simulink model "HMC"  (R2026a)
settings: Solver=ode1  StopTime=inf  FixedStep=0.0001
PreLoadFcn:
  | %load('C:\Users\bme_master\Desktop\mot\mot_6_deneme.mat')
  | 
  | 
  | %load('C:\Users\bme_master\Desktop\mot\PRE_G''s.mat')
PostLoadFcn:
  | , if any(exist('dsrtsu_mdlpostloadfcn', 'file') ~= 0), dsrtsu_mdlpostloadfcn('Execute', bdroot); end,
InitFcn:
  | %motor_control_init_m
  | %clear all
  | %close all
  | %clc
  | b=1e-8
  | StepSize = 1e-4;
  | N=1e-17;
  | 
  | VLV_0 =0;%120; %120
  | VA_0 = 0;%300; %300
  | VRV_0 = 0;%130;
  | VP_0 = 0;%500;
  | VLA_0 = 0;%20;
  | VV_0=5000;
  | VRA_0=0;
  | 
  | 
  | QLV_0 = 0;
  | QLA_0 = 0;
  | QP_0 = 0;
  | 
  | bh = 0;
  | th =0;
  | 
  | X_0 = [VLV_0 VA_0 VV_0 VP_0  VLA_0  VRA_0 VRV_0];
  | 
  | 
  | V0 = 10;
  | 
  | K1=.0004;%0.0001
  | K2=0.0009;%0.0009
  | KA=1;%1
  | C1=0.000000003;%0.0000003
  | lambda=6000;%3000
  | X_00 = [VLV_0 VA_0 VV_0 VRV_0];
  | 
  | r2 = 0.05/2;
  | A2 = pi*r2^2;
  | h2 = 0.63;
  | V2 = A2*h2;
  | 
  | 
  | r3 = 0.05/2;
  | A3 = pi*r3^2;
  | h3 = 0.63;
  | V3 = A3*h3;
  | 
  | 
  | rho = 997;
  | gg = 9.81;
  | %
  | init_min=0;
  | init_max=0;
  | %
  | PWM_Period =  StepSize;
  | PWM_Period_g1 = PWM_Period;
  | PWM_Period_g2 =PWM_Period;
  | PWM_Period_g3 = PWM_Period;
  | PWM_Period_g4 = PWM_Period;
  | PWM_Period_g5 = PWM_Period;
  | ... (+158 lines)
undefined symbols (not defined in the file or in its folder): Continuous, DiscIntNeverNeededParam, Time
libraries: powerlib_meascontrol x19, simulink x15, rti1202lib_adc_class1 x11, cstblocks x10, rti1202lib_dio_class1 x8, dspstat3 x3, rti1202lib_dac_class1 x1, dspswit3 x1, ctrlSharedLib x1, slpidlib x1, dsparch4 x1
(part 2 of 5)

== system HMC/DP_calc ==
  Subtract : Sum  Inputs=+-
  Out1 : Outport  VectorParamsAs1DForOutWhenUnconnected=off
  wires:
  [P2_mmHg] -> Subtract/1
  [P3_mmHg] -> Subtract/2
  Subtract/1 -> Out1/1

== system HMC/DV_calc ==
  DV : Scope
      settings: DataLoggingVariableName=ScopeData7
  MATLAB Function3 : MATLAB Function  TreatAsAtomicUnit=on
  Transfer Fcn1 : TransferFcn  Numerator=[100^2]  Denominator=[1 2*5*100 100^2]
  V2 : Scope
      settings: DataLoggingVariableName=ScopeData5
  V3 : Scope
      settings: DataLoggingVariableName=ScopeData6
  Out1 : Outport  VectorParamsAs1DForOutWhenUnconnected=off
  wires:
  [P2_Pa] -> MATLAB Function3/1(P2)
  MATLAB Function3/1(V2) -> V2/1
  [P3_Pa] -> MATLAB Function3/3(P3)
  [P2p_Pa] -> MATLAB Function3/2(Pp2)
  MATLAB Function3/2(V3) -> V3/1
  [P3p_Pa] -> MATLAB Function3/4(Pp3)
  MATLAB Function3/3(DV) -> Transfer Fcn1/1
  Transfer Fcn1/1 -> DV/1, Out1/1

== system HMC/IBS_LVAD ==
  Subsystem1 : Subsystem
  Unit Delay : UnitDelay  SampleTime=-1
  W : Outport  VectorParamsAs1DForOutWhenUnconnected=off
  tag scope: VAD_real=global
  wires:
  [x_pre_1] -> Subsystem1/11(VLV)
  [VAD] -> Subsystem1/10(QVAD)
  Unit Delay/1 -> [VAD_real]
  [gLV] -> Subsystem1/18(gLV)
  [PA] -> Subsystem1/20(PA1)
  Subsystem1/1(VAD) -> Unit Delay/1
  [eLV] -> Subsystem1/15(eLV)
  [eRA] -> Subsystem1/12(eRA)
  [QA] -> Subsystem1/7(QA)
  [PA] -> Subsystem1/2(PA)
  [PLV] -> Subsystem1/19(PLV1)
  [eV] -> Subsystem1/14(eV)
  [PRA] -> Subsystem1/4(PRA)
  [eAO] -> Subsystem1/13(eA)
  [gAO] -> Subsystem1/16(gA)
  [QV] -> Subsystem1/8(QV)
  [gV] -> Subsystem1/17(gV)
  [QLV] -> Subsystem1/6(QLV)
  [PV] -> Subsystem1/3(PV)
  [QLA] -> Subsystem1/5(QLA)
  [PLV] -> Subsystem1/1(PLV)
  [QRA] -> Subsystem1/9(QRA)
  Subsystem1/2(W) -> W/1

== system HMC/KALMAN 3 STATES PLA ==
  Constant7 : Constant  Value=[1 0 0;0 1 0]
  Constant8 : Constant  Value=[0;0]  VectorParams1D=off
  Demux5 : Demux  Outputs=3
  Derivative : Derivative
  Kalman Filter : ctrlSharedLib/Kalman Filter  TimeDomain=Continuous-Time  UseCurrentEstimator=on  ModelSource=Input port  ModelSourceVariable=ss(0.95,1,1,0,1)  A=0.95  B=1  C=1  D=0  NumberOfStates=3  NumberOfInputs=1  NumberOfOutputs=2  InitialEstimateSource=Dialog  X0=[100 0 0]  P0=[1e-2 1e-2 1e-5]  UseK=off  UseGH=off  NumberOfProcessNoiseInputs=1  G=1  TimeInvariantG=on  H=0  TimeInvariantH=on  Q=[100 100 1e-5]  TimeInvariantQ=on  R=[1e-6 1e-5]  TimeInvariantR=on  N=0  TimeInvariantN=on  AddInputPort=on  AddEnablePort=off  OutputEstimatedY=off  OutputP=off  Ts=-1
  MATLAB Function1 : MATLAB Function  TreatAsAtomicUnit=on
  MATLAB Function9 : MATLAB Function  TreatAsAtomicUnit=on
  Mux5 : Mux  Inputs=2
  Mux6 : Mux  Inputs=7
  Scope10 : Scope  NumInputPorts=2
      settings: ActiveDisplayYMinimum=50.21546  ActiveDisplayYMaximum=84.01485
  Scope12 : Scope  NumInputPorts=2
      settings: ActiveDisplayYMinimum=-39.55497  ActiveDisplayYMaximum=141.8795  DataLoggingVariableName=ScopeData2
  Scope13 : Scope  NumInputPorts=2
      settings: ActiveDisplayYMinimum=10.94345  ActiveDisplayYMaximum=14.67296  DataLoggingVariableName=ScopeData3
  Output : Outport  VectorParamsAs1DForOutWhenUnconnected=off
  wires:
  [PA] -> Scope10/2
  Demux5/3 -> Scope13/1, [estPLA], Output/1  "EST PLA"
  Mux5/1 -> Kalman Filter/2
  [PLA] -> Scope13/2
  [eLA] -> Mux6/6
  [PLV] -> Mux5/2
  MATLAB Function9/1(y) -> Kalman Filter/4
  Constant8/1 -> Kalman Filter/6
  [eAO] -> Mux6/4
  [eLV] -> Derivative/1, Mux6/1
  [PA] -> Mux5/1
  Mux6/1 -> MATLAB Function9/1(u), MATLAB Function1/1(u)
  [estPLA] -> MATLAB Function1/3(pla)
  [gLA] -> Mux6/7
  [V0] -> Kalman Filter/1
  Derivative/1 -> Mux6/2
  Demux5/1 -> Scope10/1
  Constant7/1 -> Kalman Filter/5
  Demux5/2 -> Scope12/1
  MATLAB Function1/1(y) -> Kalman Filter/3
  [PLV] -> MATLAB Function1/2(plv)
  [gLV] -> Mux6/3
  Kalman Filter/1 -> Demux5/1
  [PLV] -> Scope12/2
  [gAO] -> Mux6/5

== system HMC/RTI Data ==
  RTI Data Store : Subsystem  Tag=struct('private',struct('version',struct('dsVer',uint32(2)),'access',struct('modified',['21-Nov-2025 12:44:49'],'type','Model','isPerm',1)))  mask(RTI_DATA_STORE){}
      mask help:
      | RTI Data Store Block. This block is used by RTI to store internal model dependent data. Deleting this block will result in data loss.
      |
      | NEVER DELETE, COPY, OR MODIFY THIS BLOCK!
      mask Help:
      | RTI Data Store Block. This block is used by RTI to store internal model dependent data. Deleting this block will result in data loss.
      | 
      | NEVER DELETE, COPY, OR MODIFY THIS BLOCK!
      mask Display: text(0.5, 0.5, ' ', 'HorizontalAlignment', 'center');

== system HMC/Real_IBS ==
  A1 : Constant  Value=0.000234
  A2 : Constant  Value=500
  A3 : Constant  Value=1249
  A4 : Constant  Value=62584000
  Add : Sum
  Add1 : Sum  Inputs=+-
  Constant : Constant  Value=0.3682
  Delta_P1 : Gain
  EQ : Subsystem  Commented=on
  EV_int_scope : Scope
      settings: DataLoggingVariableName=ScopeData4
  EV_scope : Scope
      settings: DataLoggingVariableName=ScopeData5
  Gain : Gain  Gain=1/24
  Gain1 : Gain  Gain=0.0001
  Integrator1 : Integrator  ExternalReset=rising
  J : Constant  Value=1E-05
  K3 : Constant  Value=0.001
  K4 : Constant  Value=0.001
  KV : Constant  Value=20
  MATLAB Function1 : MATLAB Function  TreatAsAtomicUnit=on
  Memory : Memory  InitialCondition=1
  Mux1 : Mux
  Q_vad_dot1 : Subsystem  Commented=on
  Referance_Delta_V_dot : Constant  Value=0
  Subsystem2 : Subsystem
  Subsystem3 : Subsystem  Commented=on
  Subtract : Sum  Inputs=+-
  Transfer Fcn : TransferFcn  Numerator=[100^2]  Denominator=[1 2*5*100 100^2]
  Transfer Fcn1 : TransferFcn  Numerator=[100^2]  Denominator=[1 2*5*100 100^2]
  alpha_P : Constant  Value=2.34E-07
  alpha_Q : Constant  Value=2E-05
  kv : Constant  Value=0.001
  lambda : Constant  Value=0.1
  y_Scope : Scope
      settings: ActiveDisplayYMinimum=-7.21272180033628E+9  ActiveDisplayYMaximum=8.0141354018687E+8  DataLoggingVariableName=ScopeData3
  Out1 : Outport  VectorParamsAs1DForOutWhenUnconnected=off
  wires:
  MATLAB Function1/1(v) -> Gain/1, y_Scope/1
  Gain/1 -> Transfer Fcn/1
  [C_on_off] -> Integrator1/2
  Integrator1/1 -> EV_int_scope/1, MATLAB Function1/10(EV_int)
  Subsystem2/1(Out1) -> Transfer Fcn1/1
  Delta_P1/1 -> MATLAB Function1/7(DP)
  kv/1 -> MATLAB Function1/6(kv)
  KV/1 -> MATLAB Function1/5(KV)
  lambda/1 -> MATLAB Function1/4(lambda)
  J/1 -> MATLAB Function1/3(J)
  alpha_P/1 -> MATLAB Function1/2(alpha_P)
  alpha_Q/1 -> MATLAB Function1/1(alpha_Q)
  [P3_mmHg] -> Subtract/2
  Constant/1 -> Add/2
  Add/1 -> Delta_P1/1
  [P2_mmHg] -> Subtract/1
  Subtract/1 -> Add/1
  Memory/1 -> Add1/2
  [Qvad_kalman] -> Add1/1, Memory/1
  Add1/1 -> Gain1/1
  Gain1/1 -> MATLAB Function1/8(Q_vad_dot)
  K3/1 -> MATLAB Function1/11(K3)
  K4/1 -> MATLAB Function1/12(K4)
  [Qvad_kalman] -> MATLAB Function1/14(Q_vad)
  [Qgp_kalman] -> MATLAB Function1/15(Q_gp)
  Referance_Delta_V_dot/1 -> MATLAB Function1/13(DV_dot_ref)
  A1/1 -> Mux1/1
  Mux1/1 -> MATLAB Function1/16(A)
  A2/1 -> Mux1/2
  A3/1 -> Mux1/3
  A4/1 -> Mux1/4
  Transfer Fcn/1 -> Out1/1
  Transfer Fcn1/1 -> EV_scope/1, Integrator1/1, MATLAB Function1/9(EV)

== system HMC/Reference CVSs ==
  Exercise_On_Off : Constant  Value=0
  Gain1 : Gain  Gain=1/16.666
  HEART RATE : Constant  Value=60
  HeartRate : Subsystem
  Heart_Failure_On_Off : Constant  Value=0
  Non_exercise_HR(60-90) : Constant  Value=60
  PAO : Scope
      settings: ActiveDisplayYMinimum=75.8800282877439  ActiveDisplayYMaximum=129.69375884129283
  PLV : Scope
      settings: ActiveDisplayYMinimum=10.398415522297556  ActiveDisplayYMaximum=126.54338860281534  DataLoggingVariableName=ScopeData2
  Pm : Subsystem
  Pressures Flows and Volumes : Subsystem
  Product : Product
  QVAD : Subsystem
  Reset : Subsystem
  Saturation1 : Saturate  UpperLimit=500  LowerLimit=-100
  Scope : Scope
      settings: ActiveDisplayYMinimum=-1  ActiveDisplayYMaximum=1  DataLoggingVariableName=ScopeData3
  VAD_FB : Constant  Value=0
  eLV : Subsystem
  eRV : Subsystem
  PA_ref : Outport  VectorParamsAs1DForOutWhenUnconnected=off
  PLV_ref : Outport  Port=2  VectorParamsAs1DForOutWhenUnconnected=off
  QLV : Outport  Port=3  VectorParamsAs1DForOutWhenUnconnected=off
  QLA : Outport  Port=4  VectorParamsAs1DForOutWhenUnconnected=off
  tag scope: Exercise_On_Off=global, HR=global, Heart_Failure_On_Off=global, Non_exercise_HR=global, QVAD=global
  wires:
  Exercise_On_Off/1 -> [Exercise_On_Off]
  Non_exercise_HR(60-90)/1 -> [Non_exercise_HR]
  Heart_Failure_On_Off/1 -> [Heart_Failure_On_Off]
  HEART RATE/1 -> [HR]
  Product/1 -> Scope/1, [QVAD]
  VAD_FB/1 -> Product/2
  Pressures Flows and Volumes/4(RLV) -> eRV/2(VRV)
  eRV/1(eRV1) -> Pressures Flows and Volumes/4(erv1), Pressures Flows and Volumes/2(erv)
  HeartRate/1(Out1) -> eRV/1(HR), eLV/2(HR)
  eLV/1(elv) -> Pressures Flows and Volumes/3(elv1), Pressures Flows and Volumes/1(elv)
  Pressures Flows and Volumes/1(VLV) -> Saturation1/1
  Pressures Flows and Volumes/3(PLV) -> PLV/1, PLV_ref/1
  Pressures Flows and Volumes/2(PA) -> PAO/1, PA_ref/1
  Pressures Flows and Volumes/6(QLA) -> QLA/1
  Pressures Flows and Volumes/5(QLV) -> QLV/1
  [VAD_real] -> Gain1/1
  [Qvad_kalman] -> Product/1
  Saturation1/1 -> eLV/1(VLV)

== system HMC/Subsystem ==
  Input : Inport
  Clock3 : Clock
  Constant : Constant
  Divide : Product  Inputs=*/
  Gain : Gain
  Gain1 : Gain  Gain=15
  MATLAB Function : MATLAB Function  TreatAsAtomicUnit=on
  MATLAB Function1 : MATLAB Function  TreatAsAtomicUnit=on
  MATLAB Function10 : MATLAB Function  TreatAsAtomicUnit=on
  MATLAB Function9 : MATLAB Function  TreatAsAtomicUnit=on
  Moving Average : dspstat3/Moving Average  Method=Sliding window  ForgettingFactorPort=off  SpecifyWindowLength=on  WindowLength=800  ForgettingFactor=0.6  SimulateUsing=Code generation
  Unit Delay{,1..9} (10 alike) : UnitDelay  SampleTime=-1
  Out1 : Outport  VectorParamsAs1DForOutWhenUnconnected=off
  wires:
  MATLAB Function/1(lol) -> Gain1/1, Unit Delay1/1
  MATLAB Function10/1(th) -> Unit Delay6/1, MATLAB Function/1(u), Unit Delay/1
  Gain1/1 -> Moving Average/1
  MATLAB Function9/1(output) -> MATLAB Function10/2(on_off)
  Clock3/1 -> MATLAB Function10/1(time)
  Unit Delay6/1 -> MATLAB Function10/3(tpr)
  Unit Delay/1 -> MATLAB Function/2(delayed_u)
  Unit Delay1/1 -> MATLAB Function/3(pre_bob)
  Unit Delay2/1 -> MATLAB Function9/2(pwm_delayed)
  Input/1 -> Unit Delay2/1, MATLAB Function9/1(pwm)
  Moving Average/1 -> Out1/1
  Unit Delay4/1 -> MATLAB Function1/2(d_2), Unit Delay5/1
  Unit Delay5/1 -> Unit Delay7/1, MATLAB Function1/3(d_3)
  Unit Delay8/1 -> MATLAB Function1/5(d_5)
  Unit Delay7/1 -> Unit Delay8/1, MATLAB Function1/4(d_4)
  Gain/1 -> Divide/2
  Constant/1 -> Divide/1
  Unit Delay9/1 -> MATLAB Function1/6(ty)
  MATLAB Function1/1(y) -> Unit Delay9/1, Gain/1
  Unit Delay3/1 -> MATLAB Function1/1(d_1), Unit Delay4/1

== system HMC/Subsystem1 ==
  Qvad : Inport
  DP : Inport  Port=2
  "DV " : Inport  Port=3
  Derivative2 : Derivative
  Derivative3 : Derivative
  Integrator : Integrator  InitialCondition=-1.0238
  Integrator1 : Integrator  InitialCondition=-3.18e-06
  Integrator2 : Integrator  InitialCondition=247.098
  Integrator3 : Integrator  InitialCondition=-50.2777
  Integrator4 : Integrator  InitialCondition=-333.3333
  Integrator7 : Integrator  InitialCondition=694.4444
  Integrator8 : Integrator  InitialCondition=80
  Integrator9 : Integrator  InitialCondition=0.4
  MATLAB Function2 : MATLAB Function  TreatAsAtomicUnit=on
  Saturation : Saturate  UpperLimit=24  LowerLimit=0
  Scope11 : Scope
      settings: ActiveDisplayYMinimum=-0.19291  ActiveDisplayYMaximum=9.44398  DataLoggingVariableName=ScopeData2
  gam{1..6} (6 alike) : Constant  Value=5
  k1 : Constant  Value=200
  k2 : Constant  Value=200
  k3 : Constant  Value=2000
  "phi2 " : Scope  NumInputPorts=2
      settings: ActiveDisplayYMinimum=12.23414  ActiveDisplayYMaximum=110.55432  DataLoggingVariableName=ScopeData4
  phi3 : Scope  NumInputPorts=2
      settings: ActiveDisplayYMinimum=-6.23903  ActiveDisplayYMaximum=5.72515
  u : Scope
      settings: ActiveDisplayYMinimum=-1.51252  ActiveDisplayYMaximum=13.61271  DataLoggingVariableName=ScopeData3
  Out1 : Outport  VectorParamsAs1DForOutWhenUnconnected=off
  wires:
  MATLAB Function2/11(i_dot) -> Integrator9/1
  DP/1 -> Derivative3/1, MATLAB Function2/9(DP)
  Integrator9/1 -> MATLAB Function2/13(i)
  MATLAB Function2/10(W_dot) -> Integrator8/1
  MATLAB Function2/4(g4h_dot) -> Integrator3/1
  Integrator7/1 -> MATLAB Function2/6(g6h)
  Saturation/1 -> Out1/1, u/1
  MATLAB Function2/3(g3h_dot) -> Integrator2/1
  k1/1 -> MATLAB Function2/14(k1)
  Integrator4/1 -> MATLAB Function2/5(g5h)
  Integrator2/1 -> MATLAB Function2/3(g3h)
  MATLAB Function2/6(g6h_dot) -> Integrator7/1
  gam4/1 -> MATLAB Function2/20(gam4)
  gam1/1 -> MATLAB Function2/17(gam1)
  gam5/1 -> MATLAB Function2/21(gam5)
  [W] -> "phi2 "/2
  gam3/1 -> MATLAB Function2/19(gam3)
  MATLAB Function2/5(g5h_dot) -> Integrator4/1
  Integrator3/1 -> MATLAB Function2/4(g4h)
  MATLAB Function2/2(g2h_dot) -> Integrator/1
  k3/1 -> MATLAB Function2/16(k3)
  gam2/1 -> MATLAB Function2/18(gam2)
  [i] -> phi3/2
  MATLAB Function2/7(phi2) -> "phi2 "/1
  Qvad/1 -> Derivative2/1, MATLAB Function2/7(Qvad)
  Integrator/1 -> MATLAB Function2/2(g2h)
  k2/1 -> MATLAB Function2/15(k2)
  MATLAB Function2/9(u) -> Scope11/1, Saturation/1
  "DV "/1 -> MATLAB Function2/11(DV)
  Derivative2/1 -> MATLAB Function2/8(Qvad_dot)
  Integrator8/1 -> MATLAB Function2/12(W)
  Integrator1/1 -> MATLAB Function2/1(g1h)
  Derivative3/1 -> MATLAB Function2/10(DP_dot)
  MATLAB Function2/1(g1h_dot) -> Integrator1/1
  gam6/1 -> MATLAB Function2/22(gam6)
  MATLAB Function2/8(phi3) -> phi3/1

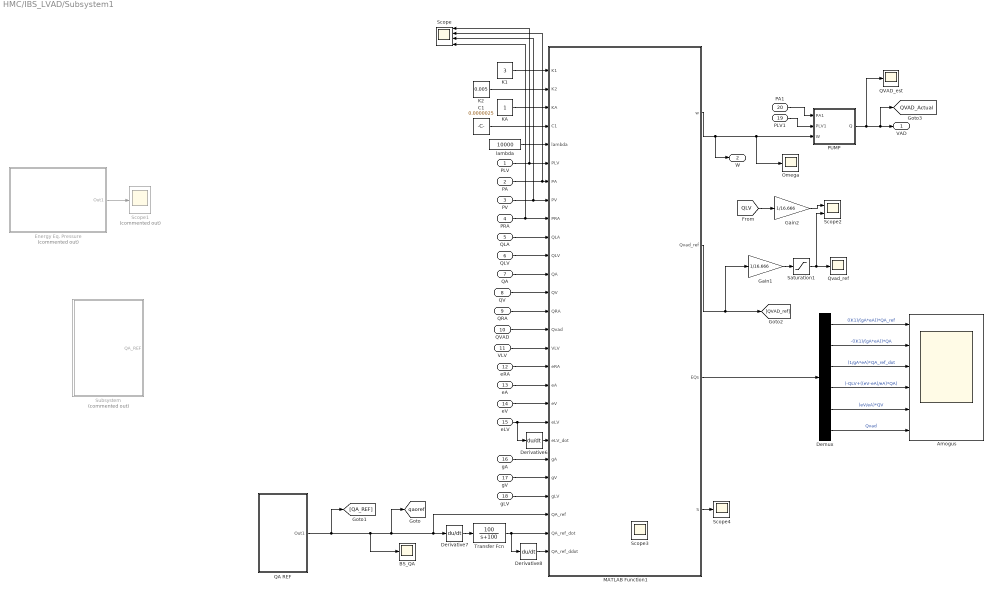
== system HMC/IBS_LVAD/Subsystem1 ==
  PLV : Inport
  PA : Inport  Port=2
  PV : Inport  Port=3
  PRA : Inport  Port=4
  QLA : Inport  Port=5
  QLV : Inport  Port=6
  QA : Inport  Port=7
  QV : Inport  Port=8
  QRA : Inport  Port=9
  QVAD : Inport  Port=10
  VLV : Inport  Port=11
  eRA : Inport  Port=12
  eA : Inport  Port=13
  eV : Inport  Port=14
  eLV : Inport  Port=15
  gA : Inport  Port=16
  gV : Inport  Port=17
  gLV : Inport  Port=18
  PLV1 : Inport  Port=19
  PA1 : Inport  Port=20
  Amogus : Scope  NumInputPorts=6
      settings: ActiveDisplayYMinimum=-45.85221  ActiveDisplayYMaximum=156.40484
  BS_QA : Scope
      settings: ActiveDisplayYMinimum=42.60777  ActiveDisplayYMaximum=71.32052
  C1 : Constant  Value=0.0000025
  Demux : Demux  Outputs=6
  Derivative6 : Derivative
  Derivative7 : Derivative
  Derivative8 : Derivative
  Energy Eq. Pressure : Subsystem  Commented=on
  Gain1 : Gain  Gain=1/16.666
  Gain2 : Gain  Gain=1/16.666
  K1 : Constant  Value=3
  K2 : Constant  Value=0.005
  KA : Constant
  MATLAB Function1 : MATLAB Function  TreatAsAtomicUnit=on
  Omega : Scope
      settings: ActiveDisplayYMinimum=-6052.53847  ActiveDisplayYMaximum=54472.84626
  PUMP : Subsystem
  QA REF : Subsystem
  QVAD_est : Scope
      settings: ActiveDisplayYMinimum=-1.6258885458551316E+197  ActiveDisplayYMaximum=1.4632996912696189E+198  DataLoggingVariableName=ScopeData3
  Qvad_ref : Scope
      settings: ActiveDisplayYMinimum=-4.125  ActiveDisplayYMaximum=17.125  DataLoggingVariableName=ScopeData2
  Saturation1 : Saturate  UpperLimit=15  LowerLimit=-2
  Scope : Scope  NumInputPorts=4
      settings: ActiveDisplayYMinimum=-6.64373  ActiveDisplayYMaximum=80.89113
  Scope1 : Scope  Commented=on
      settings: ActiveDisplayYMinimum=-18.64274  ActiveDisplayYMaximum=167.78462
  Scope2 : Scope  NumInputPorts=2
      settings: ActiveDisplayYMinimum=-8.64053  ActiveDisplayYMaximum=57.76475
  Scope3 : Scope  NumInputPorts=4
      settings: ActiveDisplayYMinimum=-22.64924  ActiveDisplayYMaximum=87.16525  DataLoggingVariableName=ScopeData3
  Scope4 : Scope
      settings: ActiveDisplayYMinimum=-1.576124585107832E+10  ActiveDisplayYMaximum=1.0457495564080603E+11  DataLoggingVariableName=ScopeData4
  Subsystem : Subsystem  Commented=on
  Transfer Fcn : TransferFcn  Numerator=[100]  Denominator=[1 100]
  lambda : Constant  Value=10000
  VAD : Outport
  W : Outport  Port=2  VectorParamsAs1DForOutWhenUnconnected=off
  tag scope: QVAD_Actual=global, qaoref=global
  wires:
  Derivative6/1 -> MATLAB Function1/21(eLV_dot)
  Derivative8/1 -> MATLAB Function1/27(QA_ref_ddot)
  Derivative7/1 -> Transfer Fcn/1
  PLV/1 -> MATLAB Function1/6(PLV), Scope/1
  PA/1 -> Scope/2, MATLAB Function1/7(PA)
  PV/1 -> Scope/3, MATLAB Function1/8(PV)
  PRA/1 -> MATLAB Function1/9(PRA), Scope/4
  QLA/1 -> MATLAB Function1/10(QLA)
  QLV/1 -> MATLAB Function1/11(QLV)
  QV/1 -> MATLAB Function1/13(QV)
  QRA/1 -> MATLAB Function1/14(QRA)
  QVAD/1 -> MATLAB Function1/15(Qvad)
  VLV/1 -> MATLAB Function1/16(VLV)
  eRA/1 -> MATLAB Function1/17(eRA)
  eA/1 -> MATLAB Function1/18(eA)
  eV/1 -> MATLAB Function1/19(eV)
  eLV/1 -> MATLAB Function1/20(eLV), Derivative6/1
  gA/1 -> MATLAB Function1/22(gA)
  gV/1 -> MATLAB Function1/23(gV)
  gLV/1 -> MATLAB Function1/24(gLV)
  lambda/1 -> MATLAB Function1/5(lambda)
  C1/1 -> MATLAB Function1/4(C1)
  KA/1 -> MATLAB Function1/3(KA)
  K2/1 -> MATLAB Function1/2(K2)
  K1/1 -> MATLAB Function1/1(K1)
  Energy Eq. Pressure/1(Out1) -> Scope1/1
  PA1/1 -> PUMP/1(PA1)
  PLV1/1 -> PUMP/2(PLV1)
  QA/1 -> MATLAB Function1/12(QA)
  MATLAB Function1/1(w) -> W/1, Omega/1, PUMP/3(W)
  PUMP/1(Q) -> QVAD_est/1, [QVAD_Actual], VAD/1
  MATLAB Function1/2(Qvad_ref) -> Gain1/1, [QVAD_ref]
  MATLAB Function1/3(EQs) -> Demux/1
  Demux/1 -> Amogus/1  "((K1)/(gA*eA))*QA_ref"
  Demux/2 -> Amogus/2  "-((K1)/(gA*eA))*QA"
  Demux/3 -> Amogus/3  "(1/gA*eA)*QA_ref_dot"
  Demux/4 -> Amogus/4  "(-QLV+((eV-eA)/eA)*QA)"
  Demux/5 -> Amogus/5  "(eV/eA)*QV"
  Demux/6 -> Amogus/6  "Qvad"
  Transfer Fcn/1 -> Derivative8/1, MATLAB Function1/26(QA_ref_dot)
  Gain1/1 -> Saturation1/1
  Saturation1/1 -> Scope2/2, Qvad_ref/1
  MATLAB Function1/4(S) -> Scope4/1
  [QLV] -> Gain2/1
  Gain2/1 -> Scope2/1
  QA REF/1(Out1) -> [QA_REF], BS_QA/1, Derivative7/1, MATLAB Function1/25(QA_ref), [qaoref]

== system HMC/RTI Data/RTI Data Store ==
  RTI Data Store : Subsystem  mask(RTI_DATA_STORE){}
      mask help:
      | RTI Data Store Block. This block is used by RTI to store internal model dependent data. Deleting this block will result in data loss.
      |
      | NEVER DELETE, COPY, OR MODIFY THIS BLOCK!
      mask Help:
      | RTI Data Store Block. This block is used by RTI to store internal model dependent data. Deleting this block will result in data loss.
      | 
      | NEVER DELETE, COPY, OR MODIFY THIS BLOCK!
      mask Display: text(0.5, 0.5, ' ', 'HorizontalAlignment', 'center');

== system HMC/Real_IBS/EQ ==
  Add : Sum  Inputs=+-
  Out1 : Outport  VectorParamsAs1DForOutWhenUnconnected=off
  wires:
  Add/1 -> Out1/1
  [Qvad_kalman] -> Add/1
  [Qgp_kalman] -> Add/2

== system HMC/Real_IBS/Q_vad_dot1 ==
  Add : Sum  Inputs=+-
  Gain : Gain  Gain=0.0001
  Memory : Memory  InitialCondition=1
  Out1 : Outport  VectorParamsAs1DForOutWhenUnconnected=off
  wires:
  Add/1 -> Gain/1
  Memory/1 -> Add/2
  [Qvad_kalman] -> Add/1, Memory/1
  Gain/1 -> Out1/1

== system HMC/Real_IBS/Subsystem2 ==
  Add : Sum  Inputs=++--
  Bias : Bias  Bias=-200  SaturateOnIntegerOverflow=off
  Di : Scope
      settings: DataLoggingVariableName=ScopeData2
  Di_fil : Scope
      settings: DataLoggingVariableName=ScopeData4
  Filter : dsparch4/Biquad Filter  Tag=BlockMethodSubSystem  FilterSource=Dialog parameters  CoeffSource=Specify via dialog  FilterObject=BQF  IIRFiltStruct=Direct form II  BiQuadCoeffs=[1 0 -1 1 -1.98917730590868747 0.998122928842567481;1 0 -1 1 -1.99887682339712125 0.999502778764492561;1 0 -1 1 -1.98546167337743062 0.994382555415759817;1 0 -1 1 -1.99788239284002689 0.998508598867118402;1 0 -1 1 -1.98177747266914928 0.990665777843165785;1 0 -1 1 -1.9968869502272546 0.997513970224382263;1 0 -1 1 -1.97813081407862823 0.986978795840895984;1 0 -1 1 -1.99588953075182562 0.996517931699864246;1 0 -1 1 -1.9745277035712836 0.98332771210439851;1 0 -1 1 -1.99488916048036424 0.995519515480505768;1 0 -1 1 -1.97097404384105257 0.97971853303218126;1 0 -1 1 -1.99388485200994503 0.994517742799882809;1 0 -1 1 -1.96747563589952557 0.976157169990785056;1 0 -1 1 -1.99287559999841468 0.993511619558198333;1 0 -1 1 -1.9640381812187746 0.972649441139076254;1 0 -1 1 -1.9918603765294165 0.992500131808049857;1 0 -1 1 -1.96066728447158622 0.969201073863081963;1 0 -1 1 -1.99083812625071888 0.991482241040779533;1 0 -1 1 -1.95736845687696981 0.965817707824264904;1 0 -1 1 -1.9898077612599665 0.990456879257776923;1 0 -1 1 -1.9541471202027223 0.962504898683150367;1 0 -1 1 -1.98876815566732601 0.989422943751322226;1 0 -1 1 -1.95100861144276672 0.959268122510698706;1 0 -1 1 -1.98771813979828282 0.988379291570923524;1 0 -1 1 -1.94795818821491329 0.956112780940170492;1 0 -1 1 -1.9866564939713538 0.987324733610933092;1 0 -1 1 -1.94500103493146481 0.953044207118534992;1 0 -1 1 -1.98558194177902592 0.986258028250384444;1 0 -1 1 -1.94214226976205429 0.950067672470320423;1 0 -1 1 -1.98449314283259648 0.985177874525446584;1 0 -1 1 -1.9393869524672831 0.947188394370231945;1 0 -1 1 -1.98338868487309505 0.984082904731780284;1 0 -1 1 -1.93674009313781958 0.944411544755887844;1 0 -1 1 -1.9822670751938718 0.982971676424040042;1 0 -1 1 -1.93420666190615642 0.94174225976142889;1 0 -1 1 -1.98112673128881744 0.981842663733223486;1 0 -1 1 -1.93179159964629132 0.939185650391120119;1 0 -1 1 -1.97996597069176028 0.980694247990994361;1 0 -1 1 -1.9294998297833843 0.936746814376371084;1 0 -1 1 -1.97878299986659512 0.979524707526990945;1 0 -1 1 -1.92733627114165396 0.934430849148917608;1 0 -1 1 -1.97757590220179225 0.978332206731453602;1 0 -1 1 -1.92530585191588055 0.932242866045421392;1 0 -1 1 -1.97634262500635804 0.977114784293697802;1 0 -1 1 -1.92341352470904958 0.930188005707673016;1 0 -1 1 -1.97508096554739243 0.975870340693791194;1 0 -1 1 -1.92166428247847465 0.928271454553140973;1 0 -1 1 -1.97378855627080174 0.974596625130084049;1 0 -1 1 -1.92006317524543801 0.926498462217623997;1 0 -1 1 -1.97246284933376437 0.973291222048371596;1 0 -1 1 -1.91861532711190197 0.924874359567190774;1 0 -1 1 -1.97110110089056612 0.971951537771248764;1 0 -1 1 -1.9173259529997968 0.923404576768406593;1 0 -1 1 -1.96970035570119051 0.970574787851587129;1 0 -1 1 -1.96825743312844925 0.969157986283889716;1 0 -1 1 -1.91620037403356203 0.922094660430911595;1 0 -1 1 -1.96676891598631487 0.967697938097663357;1 0 -1 1 -1.91524403008963962 0.920950288468642131;1 0 -1 1 -1.96523114471737892 0.966191237886682708;1 0 -1 1 -1.9144624870226008 0.91997728034052173;1 0 -1 1 -1.96364022034328034 0.964634277766319936;1 0 -1 1 -1.91386143511198448 0.919181599412194461;1 0 -1 1 -1.96199202145925877 0.96302327006018118;1 0 -1 1 -1.91344667344756569 0.918569342398695809;1 0 -1 1 -1.96028224270431561 0.96135429210992962;1 0 -1 1 -1.91322407281086937 0.918146708737974215;1 0 -1 1 -1.95850646552257301 0.959623363887627145;1 0 -1 1 -1.91319950622760726 0.917919939406437568;1 0 -1 1 -1.95666027602079073 0.95782657288087214;1 0 -1 1 -1.91337873237680567 0.917895210721354382;1 0 -1 1 -1.9547394500362798 0.955960265738452053;1 0 -1 1 -1.91376721173384245 0.918078463323577232;1 0 -1 1 -1.95274023108858819 0.954021331249064852;1 0 -1 1 -1.91436982976613135 0.918475140816755853;1 0 -1 1 -1.9506597323491186 0.952007604031682164;1 0 -1 1 -1.91519049604026392 0.919089806702840351;1 0 -1 1 -1.94849649429299498 0.949918417938814375;1 0 -1 1 -1.9162315875693412 0.919925606975950938;1 0 -1 1 -1.94625122356914093 ...(+683 chars)]  ScaleValues=[0.0347947493858621407;0.0347947493858621407;0.0347535565069614361;0.0347535565069614361;0.0347125812603675185;0.0347125812603675185;0.0346718695514397837;0.0346718695514397837;0.0346314664996788604;0.0346314664996788604;0.0345914164014912706;0.0345914164014912706;0.0345517626957872748;0.0345517626957872748;0.034512547932333687;0.034512547932333687;0.0344738137427756108;0.0344738137427756108;0.0344356008142349401;0.0344356008142349401;0.0343979488653876203;0.0343979488653876203;0.0343608966249169256;0.0343608966249169256;0.0343244818122363168;0.0343244818122363168;0.0342887411203720988;0.0342887411203720988;0.0342537102008936556;0.0342537102008936556;0.0342194236507776459;0.0342194236507776459;0.0341859150010911314;0.0341859150010911314;0.0341532167073785586;0.0341532167073785586;0.0341213601416372955;0.0341213601416372955;0.0340903755857674129;0.0340903755857674129;0.0340602922263823979;0.0340602922263823979;0.0340311381508690905;0.0340311381508690905;0.0340029403445872222;0.0340029403445872222;0.0339757246891011708;0.0339757246891011708;0.0339495159613393688;0.0339495159613393688;0.0339243378335796555;0.0339243378335796555;0.0339002128741621722;0.0339002128741621722;0.0338771625488347994;0.0338771625488347994;0.033855207222639884;0.033855207222639884;0.0338343661622545824;0.0338343661622545824;0.0338146575387014564;0.0338146575387014564;0.0337960984303496276;0.0337960984303496276;0.0337787048261313852;0.0337787048261313852;0.0337624916289029978;0.0337624916289029978;0.0337474726588831708;0.0337474726588831708;0.0337336606571065484;0.0337336606571065484;0.0337210672888346372;0.0337210672888346372;0.0337097031468702596;0.0337097031468702596;0.03369957775472672;0.03369957775472672;0.0336906995696070397;0.0336906995696070397;0.0336830759851530423;0.0336830759851530423;0.0336767133339287081;0.0336767133339287081;0.0336716168896066467;0.0336716168896066467;0.0336677908688308852;0.0336677908688308852;0.0336652384327337795;0.0336652384327337795;0.0336639616880893208;0.0336639616880893208;1]  IC=0  ICnum=0  ICden=0  a0Flag=Warning  optimizeScaleValues=on  ScaleValueMode=Specify via input port (g)  roundingMode=Floor  overflowMode=off  scaleValueFracLength=14  denProdOutputFracLength=30  denAccumFracLength=30  secondMemoryFracLength=15
      settings: SourceProductName=DSP System Toolbox
  Gain : Gain  Gain=1.33
  Gain1 : Gain  Gain=0.015625
  Gain8 : Gain  Gain=0.2008
  Gain9 : Gain  Gain=133.32
  Subtract1 : Sum  Inputs=+-
  Subtract2 : Sum  Inputs=+-
  Transfer Fcn : TransferFcn  Numerator=[100^2]  Denominator=[1 2*5*100 100^2]
  bias120 : Constant  Value=-7
  cm3 : Scope
      settings: DataLoggingVariableName=ScopeData3
  cm_h_Error : Scope
  cm_h_Error_f : Scope
      settings: DataLoggingVariableName=ScopeData2
  Out1 : Outport  VectorParamsAs1DForOutWhenUnconnected=off
  wires:
  bias120/1 -> Add/4
  Filter/1 -> Di_fil/1
  Subtract2/1 -> Add/1
  Gain/1 -> Di/1, Filter/1
  Gain8/1 -> Bias/1
  Subtract1/1 -> Add/3
  Gain9/1 -> Gain8/1
  Add/1 -> Gain9/1, Gain/1
  [P2p_mmHg] -> Subtract2/2
  [P2_mmHg] -> Subtract2/1
  [P3p_mmHg] -> Subtract1/2
  [P3_mmHg] -> Subtract1/1
  Bias/1 -> Out1/1, Gain1/1, cm3/1
  Gain1/1 -> Transfer Fcn/1, cm_h_Error/1
  Transfer Fcn/1 -> cm_h_Error_f/1

== system HMC/Real_IBS/Subsystem3 ==
  Add : Sum
  Constant : Constant  Value=0.3682
  Subtract : Sum  Inputs=+-
  Out1 : Outport  VectorParamsAs1DForOutWhenUnconnected=off
  wires:
  Add/1 -> Out1/1
  [P3_mmHg] -> Subtract/2
  [P2_mmHg] -> Subtract/1
  Subtract/1 -> Add/1
  Constant/1 -> Add/2

== system HMC/Reference CVSs/HeartRate ==
  Display : Display
  Display1 : Display
  Display2 : Display
  Switch2 : Switch  Criteria=u2 > Threshold  SaturateOnIntegerOverflow=off  InputSameDT=off
  Out1 : Outport
  tag scope: insan=global
  wires:
  [HR] -> Out1/1, Switch2/1, Display/1
  [Exercise_On_Off] -> Switch2/2
  [Non_exercise_HR] -> Switch2/3, Display1/1
  Switch2/1 -> [insan], Display2/1

== system HMC/Reference CVSs/Pm ==
  note: y = -0,3333x2 + 116,67x - 5800R² = 1
  note: y = -0,0333x 2 + 11,667x - 580
  Add18 : Sum
  Add19 : Sum
  Constant20 : Constant  Value=-580
  Gain1 : Gain  Gain=1/100
  Gain2 : Gain  Gain=-0.0333
  Gain3 : Gain  Gain=11.667
  PID : Subsystem  Commented=on
  Product15 : Product
  Scope : Scope
      settings: ActiveDisplayYMinimum=3.007  ActiveDisplayYMaximum=5.007
  tag scope: PM=global
  wires:
  Add19/1 -> Gain1/1
  Gain2/1 -> Add18/1
  Gain3/1 -> Add18/2
  [HR] -> Product15/1, Product15/2, Gain3/1
  Add18/1 -> Add19/1
  Product15/1 -> Gain2/1
  Constant20/1 -> Add19/2
  Gain1/1 -> [PM], Scope/1

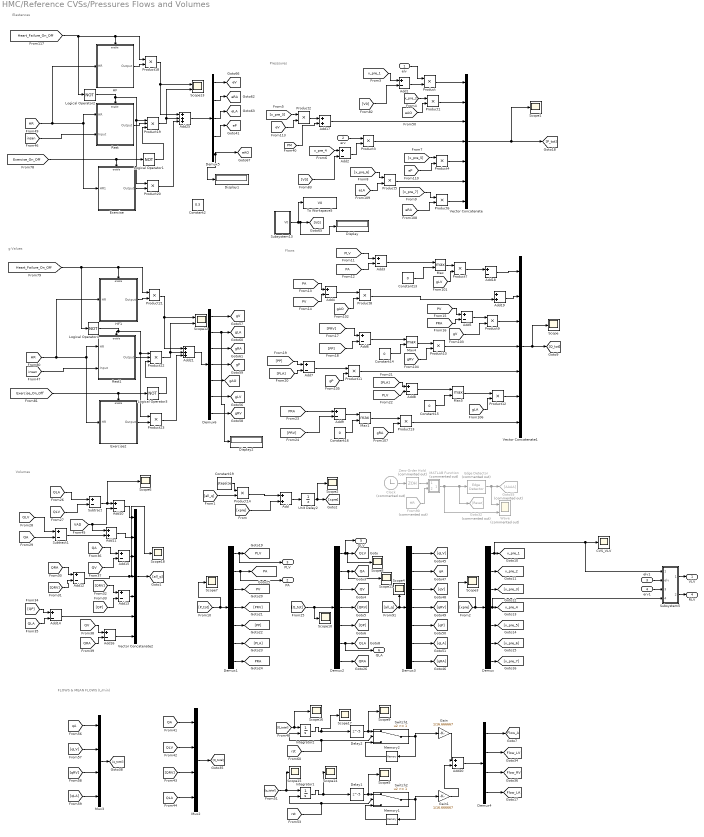
== system HMC/Reference CVSs/Pressures Flows and Volumes ==
  note: Volumes
  note: Flows
  note: Presssures
  note: g Values
  note: Elastances
  note: FLOWS & MEAN FLOWS (L/min)
  elv : Inport
  erv : Inport  Port=2
  elv1 : Inport  Port=3
  erv1 : Inport  Port=4
  Add{,11,17,19..20} (5 alike) : Sum
  Add{1..10,12..16,18} (16 alike) : Sum  Inputs=+-
  Add21 : Sum  Inputs=+++
  Add25 : Sum  Inputs=+++
  CVS_VLV : Scope
      settings: DataLoggingVariableName=ScopeData4
  Clock : Clock  Commented=on
      settings: Decimation=10000000
  Constant{13..16} (4 alike) : Constant  Value=0
  Constant19 : Constant  Value=stepsize
  Constant2 : Constant  Value=0.3
  Delay1 : Delay  DelayLength=5
  Delay2 : Delay  DelayLength=5
  Demux{,1..3,6} (5 alike) : Demux  Outputs=7
  Demux4 : Demux
  Demux5 : Demux  Outputs=5
  Display : Display
  Display1 : Display
  Display2 : Display
  Edge Detector : powerlib_meascontrol/Logic/Edge Detector  Commented=on  model=Falling  ic=0  Ts=0
      settings: SourceProductName=Simscape Electrical
  Exercise : Subsystem  TreatAsAtomicUnit=on
  Exercise2 : Subsystem  TreatAsAtomicUnit=on
  From90 : From  Commented=on  GotoTag=HR  TagVisibility=global
  Gain : Gain  Gain=1/16.666667
  Gain1 : Gain  Gain=1/16.666667
  Goto32 : Goto  Commented=on  GotoTag=Reset
  Goto55 : Goto  Commented=on  GotoTag=AAAA
  HF : Subsystem  TreatAsAtomicUnit=on
  HF1 : Subsystem  TreatAsAtomicUnit=on
  Integrator1 : Integrator  ExternalReset=either
  Integrator2 : Integrator  ExternalReset=either
  Logical Operator{1..4} (4 alike) : Logic  Operator=NOT  AllPortsSameDT=off  OutDataTypeStr=boolean
  MATLAB Function : MATLAB Function  Commented=on  TreatAsAtomicUnit=on
  Max{,1,4..5} (4 alike) : MinMax  Function=max  Inputs=2
  Memory1 : Memory  InheritSampleTime=on
  Memory2 : Memory  InheritSampleTime=on
  Mux2 : Mux
  Mux3 : Mux
  Product{,1..14,18,20..21,23} (19 alike) : Product
  Product19 : Product  Inputs=3
  Product22 : Product  Inputs=3
  Rest : Subsystem  TreatAsAtomicUnit=on
  Rest1 : Subsystem  TreatAsAtomicUnit=on
  Scope{,1..11,14..18} (17 alike) : Scope
      Scope settings: ActiveDisplayYMinimum=-77.48033  ActiveDisplayYMaximum=390.18057  DataLoggingVariableName=ScopeData3
      Scope1 settings: ActiveDisplayYMinimum=-17.90547  ActiveDisplayYMaximum=127.32097  DataLoggingVariableName=ScopeData4
      Scope10 settings: ActiveDisplayYMinimum=957.88839  ActiveDisplayYMaximum=957.93755  DataLoggingVariableName=ScopeData12
      Scope11 settings: ActiveDisplayYMinimum=-27.48687  ActiveDisplayYMaximum=51.0539  DataLoggingVariableName=ScopeData10
      Scope14 settings: ActiveDisplayYMinimum=-110.80263  ActiveDisplayYMaximum=77.31742
      Scope15 settings: ActiveDisplayYMinimum=-5789.58317  ActiveDisplayYMaximum=-2381.5007  DataLoggingVariableName=ScopeData2
      Scope16 settings: ActiveDisplayYMinimum=1027.76879  ActiveDisplayYMaximum=5015.29115  DataLoggingVariableName=ScopeData3
      Scope17 settings: ActiveDisplayYMinimum=-44.98014  ActiveDisplayYMaximum=404.82124  DataLoggingVariableName=ScopeData4
      Scope18 settings: ActiveDisplayYMinimum=2390.88881  ActiveDisplayYMaximum=2481.24108  DataLoggingVariableName=ScopeData5
      Scope2 settings: ActiveDisplayYMinimum=-34.04375  ActiveDisplayYMaximum=306.39376  DataLoggingVariableName=ScopeData3
      Scope3 settings: ActiveDisplayYMinimum=-92.27651  ActiveDisplayYMaximum=239.55796  DataLoggingVariableName=ScopeData3
      Scope4 settings: ActiveDisplayYMinimum=-3614.79854  ActiveDisplayYMaximum=3696.63533
      Scope5 settings: ActiveDisplayYMinimum=-10.26706  ActiveDisplayYMaximum=83.80402  DataLoggingVariableName=ScopeData2
      Scope6 settings: ActiveDisplayYMinimum=-1637.52208  ActiveDisplayYMaximum=5158.92158  DataLoggingVariableName=ScopeData9
      Scope7 settings: ActiveDisplayYMinimum=75.32296  ActiveDisplayYMaximum=84.1275  DataLoggingVariableName=ScopeData3
      Scope8 settings: ActiveDisplayYMinimum=-106.50454  ActiveDisplayYMaximum=958.54088  DataLoggingVariableName=ScopeData10
      Scope9 settings: ActiveDisplayYMinimum=-10.26706  ActiveDisplayYMaximum=83.80402  DataLoggingVariableName=ScopeData3
  Scope12 : Scope  NumInputPorts=2
      settings: ActiveDisplayYMinimum=-0.0275  ActiveDisplayYMaximum=0.2475  DataLoggingVariableName=ScopeData3
  Scope13 : Scope  NumInputPorts=2
      settings: ActiveDisplayYMinimum=-31.25  ActiveDisplayYMaximum=281.25  DataLoggingVariableName=ScopeData2
  Subsystem13 : Subsystem
  Subsystem5 : Subsystem
  Subtract : Sum  Inputs=+-
  Subtract1 : Sum  Inputs=+-
  Switch1 : Switch  Threshold=1  SaturateOnIntegerOverflow=off  InputSameDT=off
  Switch2 : Switch  Threshold=1  SaturateOnIntegerOverflow=off  InputSameDT=off
  To Workspace5 : ToWorkspace  VariableName=V0  SampleTime=-1
      settings: Save2DSignal=2-D array (concatenate along first dimension)
  Unit Delay2 : UnitDelay  InitialCondition=X_0  SampleTime=-1
  Vector Concatenate : Concatenate  NumInputs=7
  Vector Concatenate1 : Concatenate  NumInputs=7
  Vector Concatenate2 : Concatenate  NumInputs=7
  Wave : Scope  Commented=on  NumInputPorts=2
      settings: ActiveDisplayYMinimum=-0.125  ActiveDisplayYMaximum=1.125  DataLoggingVariableName=ScopeData2
  Zero-Order Hold : ZeroOrderHold  Commented=on  SampleTime=-1
  VLV : Outport
  PA : Outport  Port=2  VectorParamsAs1DForOutWhenUnconnected=off
  PLV : Outport  Port=3  VectorParamsAs1DForOutWhenUnconnected=off
  RLV : Outport  Port=4
  QLV : Outport  Port=5  VectorParamsAs1DForOutWhenUnconnected=off
  QLA : Outport  Port=6  VectorParamsAs1DForOutWhenUnconnected=off
  tag scope: Flow_A=global, Flow_LA=global, Flow_LV=global, Flow_RV=global, PA=global, PLV=global, PRA=global, PV=global, QA=global, QLA=global, QLV=global, QRA=global, QV=global, eAO=global, eLA=global, eP=global, eRA=global, eV=global, gAO=global, gLA=global, gLV=global, gP=global, gRA=global, gRV=global, gV=global, qA=global, x_pre_1=global, x_pre_2=global, x_pre_4=global
  wires:
  Product14/1 -> Add/1
  [xpre] -> Add/2
  elv/1 -> Product/1
  [xpre] -> Scope3/1, Demux/1
  Demux/3 -> [x_pre_3]
  Demux/5 -> [x_pre_5]
  Demux/6 -> [x_pre_6]
  Demux/7 -> [x_pre_7]
  [x_pre_1] -> Add1/1
  Add1/1 -> Product/2
  Product/1 -> Vector Concatenate/1
  Add2/1 -> Product3/2
  Product3/1 -> Vector Concatenate/4
  erv/1 -> Product3/1
  Product4/1 -> Vector Concatenate/5
  Product5/1 -> Vector Concatenate/6
  Product6/1 -> Vector Concatenate/7
  [P_tot] -> Scope7/1, Demux1/1
  Demux1/1 -> PLV/1, [PLV]
  Demux1/7 -> [PRA]
  Demux1/6 -> [PLA]
  Demux1/5 -> [PP]
  Demux1/4 -> [PRV]
  Demux1/3 -> [PV]
  [PLV] -> Add3/1
  [PA] -> Add3/2
  Max/1 -> Product7/1
  [PA] -> Add4/1
  [PV] -> Add4/2
  Add4/1 -> Product8/1
  [PV] -> Add5/1
  [PRA] -> Add5/2
  Add5/1 -> Product9/1
  Constant14/1 -> Max4/2
  [PRV] -> Add6/1
  [PP] -> Add6/2
  Max4/1 -> Product10/1
  Product10/1 -> Vector Concatenate1/4
  [PP] -> Add7/1
  [PLA] -> Add7/2
  Add7/1 -> Product11/1
  Product11/1 -> Vector Concatenate1/5
  [PLA] -> Add8/1
  [PLV] -> Add8/2
  Constant15/1 -> Max5/2
  Max5/1 -> Product12/1
  [PRA] -> Add9/1
  [PRV] -> Add9/2
  Constant16/1 -> Max1/2
  Max1/1 -> Product13/1
  Product13/1 -> Vector Concatenate1/7
  Demux2/1 -> QLV/1, Scope8/1, [QLV]
  Demux2/7 -> [QRA]
  Demux2/5 -> [QP]
  Demux2/6 -> QLA/1, [QLA]
  Demux2/3 -> [QV]
  [QLA] -> Subtract/1
  [QLV] -> Subtract1/1
  [QA] -> Subtract1/2
  [QRA] -> Add12/1
  [QRV] -> Add12/2
  [QRV] -> Add13/1
  [QP] -> Add13/2
  [QP] -> Add14/1
  [QLA] -> Add14/2
  [QA] -> Add15/1
  [QV] -> Add15/2
  Add16/1 -> Vector Concatenate2/7
  [QV] -> Add16/1
  [QRA] -> Add16/2
  Vector Concatenate/1 -> [P_tot], Scope1/1
  Vector Concatenate1/1 -> [Q_tot], Scope/1
  Vector Concatenate2/1 -> [all_q]
  [all_q] -> Product14/2
  Product2/1 -> Add17/1
  Add17/1 -> Vector Concatenate/3
  Add8/1 -> Max5/1
  Add9/1 -> Max1/1
  Add6/1 -> Max4/1
  Add3/1 -> Max/1
  Constant13/1 -> Max/2
  [x_pre_3] -> Product2/1
  [x_pre_4] -> Add2/1
  [x_pre_5] -> Product4/1
  [x_pre_6] -> Product5/1
  [x_pre_7] -> Product6/1
  Add15/1 -> Vector Concatenate2/3
  Add12/1 -> Scope18/1, Vector Concatenate2/4
  Add13/1 -> Vector Concatenate2/5
  Add14/1 -> Vector Concatenate2/6
  Constant19/1 -> Product14/1
  Add/1 -> Unit Delay2/1
  Unit Delay2/1 -> Scope2/1, [xpre]
  [Q_tot] -> Scope10/1, Demux2/1
  Product9/1 -> Vector Concatenate1/3
  [QLV] -> Subtract/2
  Clock/1 -> Zero-Order Hold/1
  Zero-Order Hold/1 -> MATLAB Function/1(u)
  Demux3/1 -> [qLV]
  Demux3/2 -> [qA]
  Demux3/3 -> [qV]
  Demux3/4 -> [qRV]
  Demux3/5 -> [qP]
  Demux3/6 -> [qLA]
  Demux3/7 -> [qRA]
  Edge Detector/1 -> Wave/1, Goto55/1
  [gLV] -> Product7/2
  [gAO] -> Product8/2
  [gV] -> Product9/2
  [gRV] -> Product10/2
  [gP] -> Product11/2
  [gLA] -> Product12/2
  [gRA] -> Product13/2
  [eRA] -> Product6/2
  [eLA] -> Product5/2
  [eP] -> Product4/2
  [V0] -> Add1/2
  [V0] -> Add2/2
  [eV] -> Product2/2
  Subtract/1 -> Scope6/1, Add10/1
  Subtract1/1 -> Add11/2
  Add10/1 -> Vector Concatenate2/1
  Add11/1 -> Vector Concatenate2/2
  Product7/1 -> Add18/1
  Add18/1 -> Vector Concatenate1/1
  Product8/1 -> Add19/2
  Add19/1 -> Vector Concatenate1/2
  Demux1/2 -> PA/1, [PA]
  MATLAB Function/1(y) -> Wave/2, Edge Detector/1, Goto32/1
  From90/1 -> MATLAB Function/2(HR)
  Demux/2 -> [x_pre_2]
  [all_q] -> Demux3/1, Scope4/1
  Demux2/4 -> [QRV]
  [VAD] -> Add11/1, Add10/2
  [PM] -> Add17/2
  Subsystem5/2(Output1) -> RLV/1
  Subsystem5/1(Out1) -> VLV/1
  Demux/4 -> Subsystem5/4(In4), [x_pre_4]
  erv1/1 -> Subsystem5/3(erv)
  elv1/1 -> Subsystem5/2(elv)
  Demux/1 -> Subsystem5/1(In1), CVS_VLV/1, [x_pre_1]
  [insan] -> Rest1/2(Input)
  HF/1(Output) -> Product18/2
  Demux5/2 -> [eRA]
  Demux6/3 -> [gRA]
  Rest1/1(Output) -> Product22/2
  Demux5/1 -> [eV]
  Exercise2/1(Output) -> Product23/2
  [Heart_Failure_On_Off] -> HF1/Enable, Product21/1, Logical Operator4/1
  Product23/1 -> Add21/3
  Logical Operator3/1 -> Product22/3
  Product20/1 -> Add25/3
  Exercise/1(Output) -> Product20/2
  Product18/1 -> Add25/1, Scope13/1
  Product22/1 -> Scope12/2, Add21/2
  Demux6/4 -> [gP]
  Demux5/4 -> [eP]
  [insan] -> Rest/2(Input)
  [Heart_Failure_On_Off] -> Logical Operator2/1, Product18/1, HF/Enable
  Demux6/1 -> [gV]
  Demux6/2 -> Display2/1, [gLA]
  HF1/1(Output) -> Product21/2
  Logical Operator4/1 -> Rest1/Enable, Product23/1, Product22/1
  Add21/1 -> Demux6/1
  Demux6/6 -> [gLV]
  [HR] -> HF/1(HR), Exercise/1(HR1), Rest/1(HR)
  Add25/1 -> Demux5/1
  [Exercise_On_Off] -> Logical Operator3/1, Exercise2/Enable
  Rest/1(Output) -> Product19/2
  Logical Operator2/1 -> Product20/1, Product19/1, Rest/Enable
  Demux6/7 -> [gRV]
  Logical Operator1/1 -> Product19/3
  Product21/1 -> Add21/1, Scope12/1
  Product19/1 -> Scope13/2, Add25/2
  [Exercise_On_Off] -> Logical Operator1/1, Exercise/Enable
  Demux5/3 -> [eLA]
  [HR] -> HF1/1(HR), Exercise2/1(HR), Rest1/1(HR)
  Subsystem13/1(V0) -> To Workspace5/1, Display/1, [V0]
  [x_pre_2] -> Product1/1
  [eAO] -> Product1/2
  Product1/1 -> Vector Concatenate/2
  Demux6/5 -> [gAO]
  Demux5/5 -> [eAO], Display1/1
  Demux2/2 -> Scope11/1, [QA]
  [rst] -> Switch1/2, Integrator2/2
  Gain/1 -> Add20/1
  [rst] -> Integrator1/2, Switch2/2
  Switch2/1 -> Gain1/1, Memory1/1
  Delay1/1 -> Switch2/1, Scope5/1
  [Q_total] -> Scope16/1, Integrator2/1
  Delay2/1 -> Scope9/1, Switch1/1
  Demux4/3 -> [Flow_RV]
  Memory1/1 -> Switch2/3
  Demux4/2 -> [Flow_LV]
  Integrator1/1 -> Scope14/1, Delay1/1
  [q_total] -> Scope15/1, Integrator1/1
  Memory2/1 -> Switch1/3
  Integrator2/1 -> Scope17/1, Delay2/1
  Gain1/1 -> Add20/2
  [QLA] -> Mux2/4
  Switch1/1 -> Memory2/1, Gain/1
  Demux4/4 -> [Flow_LA]
  Add20/1 -> Demux4/1
  [qLA] -> Mux3/4
  [QLV] -> Mux2/2
  [qA] -> Mux3/1
  [qRV] -> Mux3/3
  Mux3/1 -> [q_total]
  [qLV] -> Mux3/2
  Demux4/1 -> [Flow_A]
  Mux2/1 -> [Q_total]
  [QA] -> Mux2/1
  [QRV] -> Mux2/3
  Product12/1 -> Vector Concatenate1/6

== system HMC/Reference CVSs/QVAD ==
  Gain3 : Gain  Gain=16.666
  Product : Product
  Saturation : Saturate  UpperLimit=inf  LowerLimit=30
  Sine Wave : Sin  Amplitude=0.8  Frequency=0.4  SampleTime=0
  tag scope: VAD=global, VADQ=global
  wires:
  Gain3/1 -> [VAD], Product/1
  Sine Wave/1 -> Product/2
  Product/1 -> Saturation/1
  [QVAD] -> [VADQ], Gain3/1

== system HMC/Reference CVSs/Reset ==
  Clock2 : Clock
  Constant10 : Constant
  Constant11 : Constant  Value=0
  Constant12 : Constant  Value=10
  Mod2 : Math  Operator=mod  SignedPower=on
  Scope5 : Scope
      settings: ActiveDisplayYMinimum=-0.125  ActiveDisplayYMaximum=1.125  DataLoggingVariableName=ScopeData4
  Switch2 : Switch  Threshold=10-000001  SaturateOnIntegerOverflow=off  InputSameDT=off
  tag scope: dedect=global, rst=global
  wires:
  Mod2/1 -> Switch2/2, [dedect]
  Constant11/1 -> Switch2/3
  Switch2/1 -> Scope5/1, [rst]
  Constant10/1 -> Switch2/1
  Constant12/1 -> Mod2/2
  Clock2/1 -> Mod2/1

== system HMC/Reference CVSs/eLV ==
  VLV : Inport
  HR : Inport  Port=2
  Clock1 : Clock
  Constant : Constant  Value=3
  Display : Display
  LV_e_min : Subsystem
  Scope : Scope
      settings: ActiveDisplayYMinimum=-0.72024  ActiveDisplayYMaximum=3.41705
  Subsystem1 : Subsystem
  Switch : Switch  Criteria=u2 > Threshold  Threshold=0.9  SaturateOnIntegerOverflow=off  InputSameDT=off
  Switch1 : Switch  Criteria=u2 > Threshold  Threshold=0.9  SaturateOnIntegerOverflow=off  InputSameDT=off
  eLV1 : Subsystem
  eLVsick : Subsystem
  elv : Outport
  tag scope: eLV=global
  wires:
  Clock1/1 -> Subsystem1/4(t)
  Subsystem1/1(elv) -> Scope/1, [eLV], elv/1
  VLV/1 -> LV_e_min/1(VLV)
  HR/1 -> Subsystem1/3(HR)
  LV_e_min/1(eLV_min_O) -> Subsystem1/2(eLV_min)
  [Heart_Failure_On_Off] -> Switch/2
  Switch1/1 -> Switch/3
  Constant/1 -> Switch1/3
  [Exercise_On_Off] -> Switch1/2
  eLV1/1(Output) -> Switch1/1
  Switch/1 -> Display/1, Subsystem1/1(eLV_max)
  eLVsick/1(Output) -> Switch/1

== system HMC/Reference CVSs/eRV ==
  HR : Inport
  VRV : Inport  Port=2
  Clock2 : Clock
  Display : Display
  RV_e_min : Subsystem
  Subsystem2 : Subsystem
  Switch : Switch  Criteria=u2 > Threshold  Threshold=0.9  SaturateOnIntegerOverflow=off  InputSameDT=off
  eRV2 : Subsystem
  eRVhf : Subsystem
  eRV1 : Outport
  Out1 : Outport  Port=2
  tag scope: eRV=global
  wires:
  Clock2/1 -> Subsystem2/3(t)
  HR/1 -> Subsystem2/4(HR)
  VRV/1 -> RV_e_min/1(VRV)
  Subsystem2/1(eRV) -> Out1/1, [eRV], eRV1/1
  RV_e_min/1(eRV_min_O) -> Subsystem2/2(eRV_min)
  eRV2/1(Output) -> Switch/3
  eRVhf/1(Output) -> Switch/1
  [Heart_Failure_On_Off] -> Switch/2
  Switch/1 -> Display/1, Subsystem2/1(eRV_max)

== system HMC/IBS_LVAD/Subsystem1/Energy Eq. Pressure ==
  Clock3 : Clock
  Constant5 : Constant
  Divide : Product  Inputs=*/
  Integrator : Integrator
  Integrator1 : Integrator
  Product : Product
  Product1 : Product
  Switch3 : Switch  Criteria=u2 > Threshold  Threshold=15  SaturateOnIntegerOverflow=off  InputSameDT=off
  Out1 : Outport
  wires:
  Integrator/1 -> Divide/1
  [qaoref] -> Integrator1/1, Product/2
  Switch3/1 -> Product1/1
  Integrator1/1 -> Divide/2
  Divide/1 -> Product1/2
  Constant5/1 -> Switch3/1
  Product/1 -> Integrator/1
  Product1/1 -> Out1/1
  [PA] -> Product/1
  Clock3/1 -> Switch3/2

== system HMC/IBS_LVAD/Subsystem1/PUMP ==
  PA1 : Inport
  PLV1 : Inport  Port=2
  W : Inport  Port=3
  Add1 : Sum  Inputs=+-
  Gain : Gain  Gain=16.666
  Unit Delay2 : UnitDelay  InitialCondition=5  SampleTime=-1
  VAD1 : MATLAB Function  TreatAsAtomicUnit=on
  Q : Outport
  wires:
  Unit Delay2/1 -> VAD1/1(Q_pre)
  PLV1/1 -> Add1/2
  W/1 -> VAD1/2(W)
  PA1/1 -> Add1/1
  VAD1/1(Q) -> Gain/1, Unit Delay2/1
  Add1/1 -> VAD1/3(DP)
  Gain/1 -> Q/1

== system HMC/IBS_LVAD/Subsystem1/QA REF ==
  Add4 : Sum  Inputs=+++++
  Add5 : Sum
  Clock4 : Clock
  Constant : Constant  Value=60
  Gain Regulator : Subsystem
  Subsystem18 : Subsystem
  Subsystem19 : Subsystem
  Subsystem20 : Subsystem
  Subsystem21 : Subsystem
  Subsystem22 : Subsystem
  Switch3 : Switch  Criteria=u2 > Threshold  Threshold=9  SaturateOnIntegerOverflow=off  InputSameDT=off
  Unit Delay1 : UnitDelay  SampleTime=-1
  Out1 : Outport  VectorParamsAs1DForOutWhenUnconnected=off
  wires:
  Switch3/1 -> Unit Delay1/1
  Constant/1 -> Switch3/3
  [dedect] -> Subsystem19/1(In1), Subsystem18/1(In1), Subsystem22/1(In1), Subsystem21/1(In1), Subsystem20/1(In1)
  Subsystem20/1(Out1) -> Add4/2
  Clock4/1 -> Switch3/2
  Add4/1 -> Add5/1
  Subsystem21/1(Out1) -> Add4/3
  Subsystem22/1(Out1) -> Add4/4
  Subsystem18/1(Out1) -> Add4/5
  Subsystem19/1(Out1) -> Add4/1
  Add5/1 -> Switch3/1
  Unit Delay1/1 -> Out1/1
  Gain Regulator/1(Out1) -> Add5/2

== system HMC/IBS_LVAD/Subsystem1/Subsystem ==
  Bias2 : Bias  Bias=10  SaturateOnIntegerOverflow=off
  Constant6 : Constant  Value=60
  Constant7 : Constant  Value=0
  Constant8 : Constant
  Delay1 : Delay  DelayLength=5
  Divide : Product  Inputs=*/
  HeartRate1 : Subsystem
  Integrator1 : Integrator  ExternalReset=either
  Memory1 : Memory  InheritSampleTime=on
  Pm1 : Subsystem
  Pressures Flows and Volumes1 : Subsystem
  Scope4 : Scope  NumInputPorts=3
      settings: ActiveDisplayYMinimum=46.97802  ActiveDisplayYMaximum=99.64718  DataLoggingVariableName=ScopeData2
  Switch2 : Switch  Threshold=1-0.01  SaturateOnIntegerOverflow=off  InputSameDT=off
  Switch21 : Switch  Threshold=10-0.0005  SaturateOnIntegerOverflow=off  InputSameDT=off
  Transfer Fcn1 : TransferFcn  Numerator=[0.5]  Denominator=[1 .5]
  eLV1 : Subsystem
  eRV1 : Subsystem
  QA_REF : Outport
  tag scope: AAAA1=global, Exercise_REF=global, HR_REF=global, Non_exercise_HR_REF=global
  wires:
  Divide/1 -> Delay1/1
  [AAAA1] -> Integrator1/2, Switch2/2
  eRV1/1(eRV1) -> Pressures Flows and Volumes1/2(erv)
  Integrator1/1 -> Divide/1
  Constant6/1 -> [Non_exercise_HR_REF]
  eLV1/1(elv) -> Pressures Flows and Volumes1/1(elv)
  HeartRate1/1(Out1) -> eRV1/1(HR), eLV1/2(HR)
  Delay1/1 -> Switch2/1
  Pressures Flows and Volumes1/2(Output) -> eLV1/1(VLV)
  Pressures Flows and Volumes1/3(Output1) -> eRV1/2(VRV)
  [HR] -> [HR_REF]
  [detection] -> Switch21/2
  [Exercise_On_Off] -> [Exercise_REF]
  Constant7/1 -> Switch21/3
  Constant8/1 -> Switch21/1
  Switch2/1 -> Scope4/3, Memory1/1
  [beat_per_min] -> Divide/2
  Switch21/1 -> [AAAA1]
  Memory1/1 -> Switch2/3
  Transfer Fcn1/1 -> QA_REF/1, Scope4/1
  Bias2/1 -> Transfer Fcn1/1, Scope4/2, Integrator1/1
  Pressures Flows and Volumes1/1(QA_REF) -> Bias2/1

== system HMC/RTI Data/RTI Data Store/RTI Data Store ==
  RTI Data Store : Subsystem  mask(RTI_DATA_STORE){}
      mask help:
      | RTI Data Store Block. This block is used by RTI to store internal model dependent data. Deleting this block will result in data loss.
      |
      | NEVER DELETE, COPY, OR MODIFY THIS BLOCK!
      mask Help:
      | RTI Data Store Block. This block is used by RTI to store internal model dependent data. Deleting this block will result in data loss.
      | 
      | NEVER DELETE, COPY, OR MODIFY THIS BLOCK!
      mask Display: text(0.5, 0.5, ' ', 'HorizontalAlignment', 'center');
